simulink model "suspension_controler"  (R2020b)
settings: Solver=ode1be  StartTime=0.0  StopTime=T  FixedStep=step  RelTol=1e-3
values from neighbouring files (symbols this model uses):
  K = [0 2.3e6 5e8 0 8e6]    [parameters.m]
settings Model: Creator=kpiekorz  LastModifiedBy=kpiekorz
settings OptimizationCC: OptimizeBlockIOStorage=off  MemcpyThreshold=1024  OptimizeDataStoreBuffers=off  BusAssignmentInplaceUpdate=off
settings DebuggingCC: AlgebraicLoopMsg=error  ArtificialAlgebraicLoopMsg=error  SFUnexpectedBacktrackingDiag=warning  SFNoUnconditionalDefaultTransitionDiag=warning
settings HardwareCC: ProdBitPerLong=64  ProdHWDeviceType=Intel->x86-64 (Linux 64)
settings RTWCC: GenCodeOnly=on  GenerateReport=on  BuildConfiguration=Debug  LaunchReport=on
settings CodeAppCC: ForceParamTrailComments=on  MATLABSourceComments=on  EnableCustomComments=on
settings GRTTargetCC: CombineSignalStateStructs=on  SupportVariableSizeSignals=on  MultiInstanceErrorCode=Warning

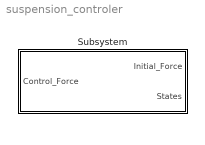
== system suspension_controler ==
  Subsystem : Subsystem

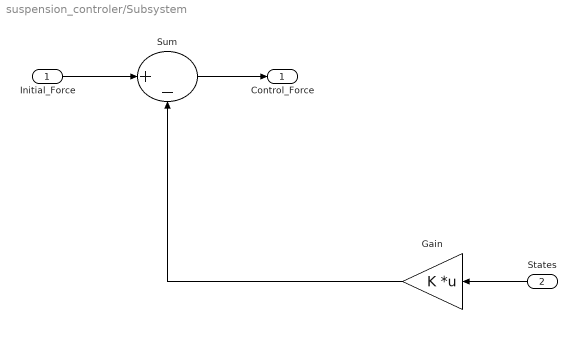
== system suspension_controler/Subsystem ==
  Initial_Force : Inport
  States : Inport  Port=2
  Gain : Gain  Gain=K  Multiplication=Matrix(K*u)
  Sum : Sum  Inputs=|+-
  Control_Force : Outport
  wires:
  Sum/1 -> Control_Force/1
  States/1 -> Gain/1
  Initial_Force/1 -> Sum/1
  Gain/1 -> Sum/2
